simulink model "count_upto_5_0_5_2016"  (R2016b)
settings: Solver=VariableStepAuto  StartTime=0.0  StopTime=10.0  FixedStep=1  MaxStep=0.2  RelTol=1e-3
settings Model: Creator=AKSHAY JP PAWAR  LastModifiedBy=AKSHAY JP PAWAR
settings DataIOCC: ReturnWorkspaceOutputs=on
settings SFSimCC: SimUseLocalCustomCode=on
settings RTWCC: RTWUseLocalCustomCode=on

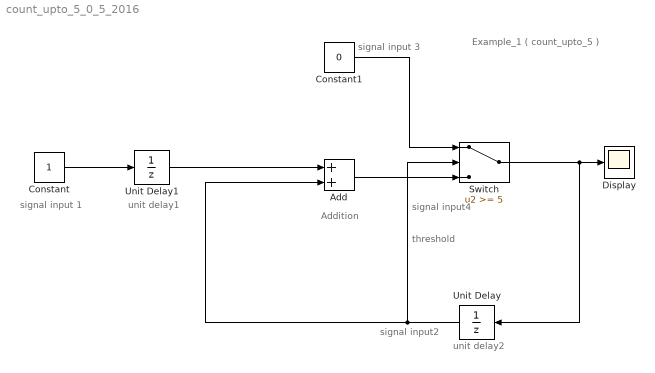
== system count_upto_5_0_5_2016 ==
  note: unit delay2
  note: signal input 3
  note: Example_1 ( count_upto_5 )
  note: signal input4
  note: threshold
  note: signal input2
  note: Addition
  note: unit delay1
  note: signal input 1
  Add : Sum
  Constant : Constant
  Constant1 : Constant  Value=0
  "Display " : Scope
  Switch : Switch  Threshold=5
  Unit Delay : UnitDelay  SampleTime=-1  HasFrameUpgradeWarning=on
  Unit Delay1 : UnitDelay  SampleTime=-1  HasFrameUpgradeWarning=on
  wires:
  Constant/1 -> Unit Delay1/1
  Unit Delay/1 -> Add/2, Switch/2
  Unit Delay1/1 -> Add/1
  Constant1/1 -> Switch/1
  Add/1 -> Switch/3
  Switch/1 -> Unit Delay/1, "Display "/1
